simulink model "problem1"  (R2020b)
settings: Solver=VariableStepAuto  StartTime=0.0  StopTime=10.0  RelTol=1e-3
PostLoadFcn:
  | k12=1
  | m2=200
settings Model: Creator=AVM  LastModifiedBy=AVM

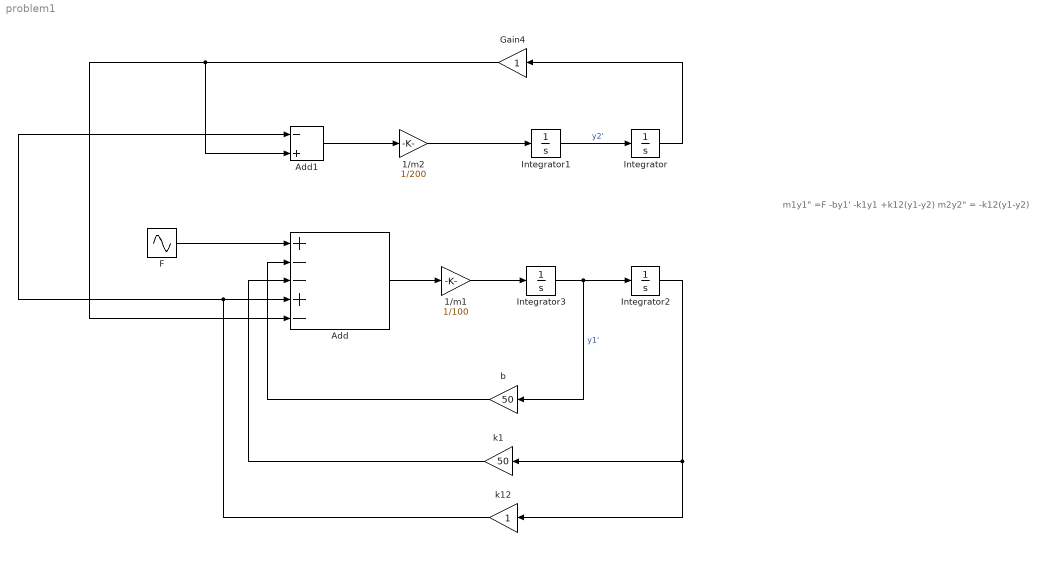
== system problem1 ==
  note: m1y1" =F -by1' -k1y1 +k12(y1-y2)
      | m2y2" = -k12(y1-y2)
  1/m1 : Gain  Gain=1/100
  1/m2 : Gain  Gain=1/200
  Add : Sum  Inputs=+--+-
  Add1 : Sum  Inputs=-+
  F : Sin  Amplitude=2  Frequency=10  SampleTime=0
  Gain4 : Gain
  Integrator{,1..3} (4 alike) : Integrator
  b : Gain  Gain=50
  k1 : Gain  Gain=50
  k12 : Gain
  wires:
  Integrator1/1 -> Integrator/1  "y2'"
  Integrator3/1 -> b/1, Integrator2/1  "y1'"
  F/1 -> Add/1
  Add/1 -> 1/m1/1
  1/m1/1 -> Integrator3/1
  b/1 -> Add/2
  Integrator2/1 -> k12/1, k1/1
  k1/1 -> Add/3
  k12/1 -> Add1/1, Add/4
  Integrator/1 -> Gain4/1
  Gain4/1 -> Add1/2, Add/5
  1/m2/1 -> Integrator1/1
  Add1/1 -> 1/m2/1
